simulink model "P2_Ex9a"  (R2018a)
settings: Solver=VariableStepAuto  StartTime=0.0  StopTime=10.0  RelTol=1e-3
PreLoadFcn:
  | % Model
  | K0=0.82/0.017;
  | tau0=0.26;
  | Kt=0.017;
  | % Sampling times
  | Tg=0.005;
  | Ts=0.01;
  | % Motor limits
  | Vmax=5;
  | Vmin=-5;
  | % Proportional controller's gain
  | Kp=1;
settings Model: Creator=Eneko Lerma  LastModifiedBy=Eneko Lerma

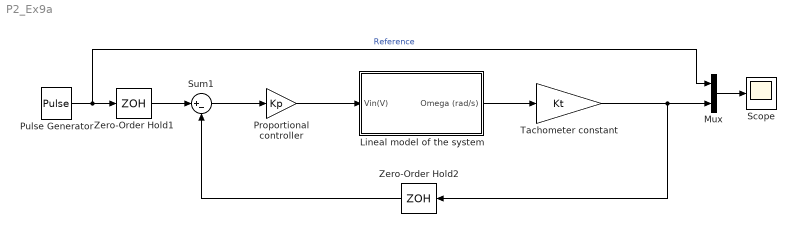
== system P2_Ex9a ==
  Lineal model of the system : Subsystem
  Mux : Mux  Inputs=2
  Proportional controller : Gain  Gain=Kp
  Pulse Generator : DiscretePulseGenerator  PulseType=Time based  Period=5  PulseWidth=50
  Scope : Scope
  Sum1 : Sum  Inputs=|+-
  Tachometer constant : Gain  Gain=Kt
  Zero-Order Hold1 : ZeroOrderHold  SampleTime=Ts
  Zero-Order Hold2 : ZeroOrderHold  SampleTime=Ts
  wires:
  Sum1/1 -> Proportional controller/1
  Pulse Generator/1 -> Mux/1, Zero-Order Hold1/1  "Reference"
  Tachometer constant/1 -> Zero-Order Hold2/1, Mux/2
  Mux/1 -> Scope/1
  Proportional controller/1 -> Lineal model of the system/1(Vin(V))
  Lineal model of the system/1(Omega (rad/s)) -> Tachometer constant/1
  Zero-Order Hold1/1 -> Sum1/1
  Zero-Order Hold2/1 -> Sum1/2

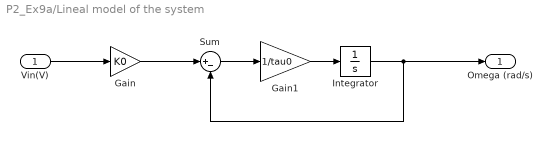
== system P2_Ex9a/Lineal model of the system ==
  Vin(V) : Inport
  Gain : Gain  Gain=K0
  Gain1 : Gain  Gain=1/tau0
  Integrator : Integrator
  Sum : Sum  Inputs=|+-
  Omega (rad/s) : Outport
  wires:
  Integrator/1 -> Omega (rad/s)/1, Sum/2
  Sum/1 -> Gain1/1
  Vin(V)/1 -> Gain/1
  Gain1/1 -> Integrator/1
  Gain/1 -> Sum/1
